simulink library "tcc"  (Simulink 8.1)
settings: Solver=ode1  StartTime=0.0  StopTime=Inf  FixedStep=0.001  RelTol=1e-3
PostLoadFcn:
  | , if any(exist('dsrtsu_mdlpostloadfcn', 'file') == [2, 3, 6]), try dsrtsu_mdlpostloadfcn('Execute', bdroot); catch fprintf('Error in PostLoadFcn (dsrtsu_mdlpostloadfcn) for model "%s":\n %s\n', bdroot, lasterr); end, end,
undefined symbols (not defined in the file or in its folder): KIFO_TTCDefault_s
libraries: simulink x4, hcu_lib x4
settings Model: DSRTSU_INTERNAL_RTI_VER=450  DSRTSU_INTERNAL_RTI_TYPE=rti1401  RTICANMMDATA=struct('GeneralSetupData',struct('modelroot','D:\PROJECTS\HAITEC\TAIWAN_HAITEC_SVN\trunk\AdasDragon\software\sw_development\arch\app\ifo','generalsettings',struct('filesettings',struct('destfolder',struct('Name','RTICANMM_FILES','Check',1),'buildfolder',struct('Name','.','Check',1),'AbsDestfolder',struct('Name','D:\PROJECTS\HAITEC\TAIWAN_HAITEC_SVN\trunk\AdasDragon\software\sw_development\arch\app\ifo\RTICANMM_FILES'),'AbsBuildfolder',struct('Name','D:\PROJECTS\HAITEC\TAIWAN_HAITEC_SVN\trunk\AdasDragon\software\sw_development\arch\app\ifo'))),'options',struct('addpaths',1,'rmpaths',1,'addtrcexclusion',logical(1),'cannavigator',struct('checkmonitoring',0),'show_usrtrc',0,'use_usrtrc',0),'advanced',struct('options',[1 1 1 1 1 1 1 1 1 1 1 1 1 1 1 1 1 1 1 1 1 1 1 1 1 1 1 1 1 1 1 1 1 1 1 1 1 1 1 1 1 1 1 1 1 1 1 1 1 1 1 1 1 1 1 1 1 1 1 1 1 1 1 1 1 1 1 1 1 1 1 1 1 1 1 1 1 1 1 1 1 1 1 1 1 1 1 1 1 1 1 1 1 1 1 1 1 1 1 1]),'MPSetup',{{}},'modelname','tcc','block','tcc'))  DSRTSU_INTERNAL_RTIFPGA=40  Creator=tescamilla  LastModifiedBy=tescamilla

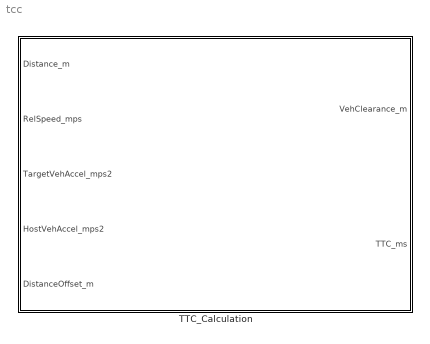
== system tcc ==
  TTC_Calculation : Subsystem

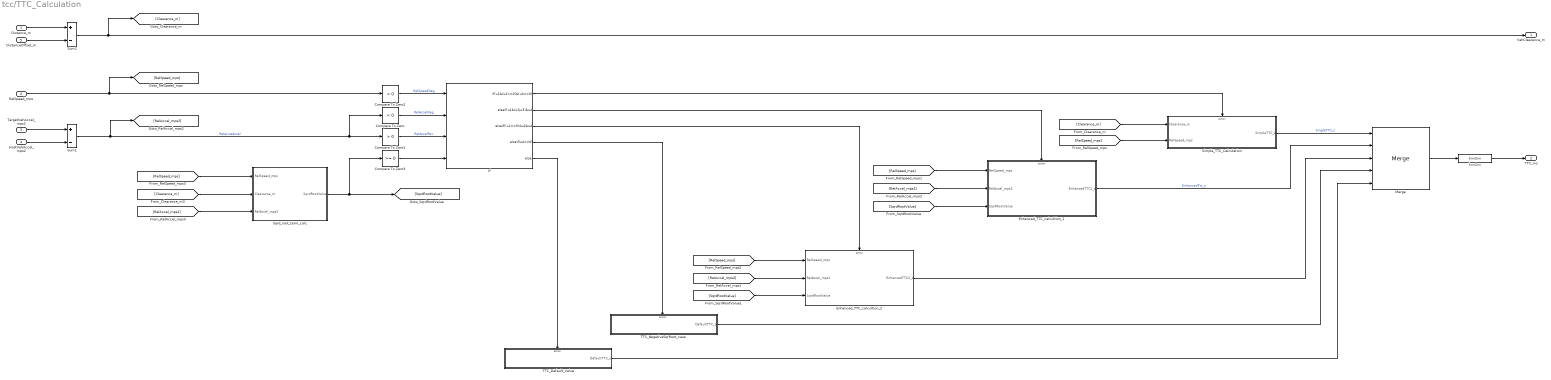
== system tcc/TTC_Calculation ==
  Distance_m : Inport
  RelSpeed_mps : Inport  Port=2
  TargetVehAccel_mps2 : Inport  Port=3
  HostVehAccel_mps2 : Inport  Port=4
  DistanceOffset_m : Inport  Port=5
  Compare To Zero : simulink/Logic and Bit Operations/Compare To Zero  relop=<  OutDataTypeStr=boolean
  Compare To Zero1 : simulink/Logic and Bit Operations/Compare To Zero  relop=>  OutDataTypeStr=boolean
  Compare To Zero2 : simulink/Logic and Bit Operations/Compare To Zero  relop=<  OutDataTypeStr=boolean
  Compare To Zero3 : simulink/Logic and Bit Operations/Compare To Zero  relop=>=  OutDataTypeStr=boolean
  Enhanced_TTC_calcultion_1 : Subsystem
  Enhanced_TTC_calcultion_2 : Subsystem
  If : If  NumInputs=4  IfExpression=u1&(u2==0)&(u3==0)  ElseIfExpressions=u1&(u2|u3)&u4,(u1==0)&u2&u4,u4==0
  Merge : Merge  Inputs=5  InitialOutput=KIFO_TTCDefault_s
  Simple_TTC_Calculation : Subsystem
  Sqrd_root_term_calc : Subsystem
  Sum1 : Sum  Inputs=+-
  Sum2 : Sum  Inputs=+-
  TTC_Default_Value : Subsystem
  TTC_NegativeSqrRoot_case : Subsystem
  kxx2xx : hcu_lib/kxx2xx
  VehClearance_m : Outport
  TTC_ms : Outport  Port=2
  wires:
  TargetVehAccel_mps2/1 -> Sum1/1
  HostVehAccel_mps2/1 -> Sum1/2
  Sum1/1 -> [RelAccel_mps2], Compare To Zero/1, Compare To Zero1/1  "RelativeAccel"
  RelSpeed_mps/1 -> [RelSpeed_mps], Compare To Zero2/1
  Compare To Zero2/1 -> If/1  "RelSpeedNeg"
  Compare To Zero/1 -> If/2  "RelAccelNeg"
  Compare To Zero1/1 -> If/3  "RelAccelPos"
  Distance_m/1 -> Sum2/1
  DistanceOffset_m/1 -> Sum2/2
  Sum2/1 -> [Clearance_m], VehClearance_m/1
  If/1 -> Simple_TTC_Calculation/Action
  If/2 -> Enhanced_TTC_calcultion_1/Action
  [Clearance_m] -> Simple_TTC_Calculation/1(Clearance_m)
  [RelSpeed_mps] -> Simple_TTC_Calculation/2(RelSpeed_mps)
  [RelSpeed_mps] -> Enhanced_TTC_calcultion_1/1(RelSpeed_mps)
  [RelAccel_mps2] -> Enhanced_TTC_calcultion_1/2(RelAccel_mps2)
  If/3 -> Enhanced_TTC_calcultion_2/Action
  [RelAccel_mps2] -> Enhanced_TTC_calcultion_2/2(RelAccel_mps2)
  [RelSpeed_mps] -> Enhanced_TTC_calcultion_2/1(RelSpeed_mps)
  If/5 -> TTC_Default_Value/Action
  Simple_TTC_Calculation/1(SimpleTTC_s) -> Merge/1  "SingleTTC_s"
  Enhanced_TTC_calcultion_1/1(EnhancedTTC1_s) -> Merge/2  "EnhancedTtc_s"
  Enhanced_TTC_calcultion_2/1(EnhancedTTC2_s) -> Merge/3
  TTC_Default_Value/1(DefaultTTC_s) -> Merge/5
  Merge/1 -> kxx2xx/1
  Compare To Zero3/1 -> If/4
  If/4 -> TTC_NegativeSqrRoot_case/Action
  TTC_NegativeSqrRoot_case/1(DefaultTTC_s) -> Merge/4
  [SqrdRootValue] -> Enhanced_TTC_calcultion_1/3(SqrdRootValue)
  [SqrdRootValue] -> Enhanced_TTC_calcultion_2/3(SqrdRootValue)
  Sqrd_root_term_calc/1(SqrdRootValue) -> Compare To Zero3/1, [SqrdRootValue]
  [RelSpeed_mps] -> Sqrd_root_term_calc/1(RelSpeed_mps)
  [Clearance_m] -> Sqrd_root_term_calc/2(Clearance_m)
  [RelAccel_mps2] -> Sqrd_root_term_calc/3(RelAccel_mps2)
  kxx2xx/1 -> TTC_ms/1

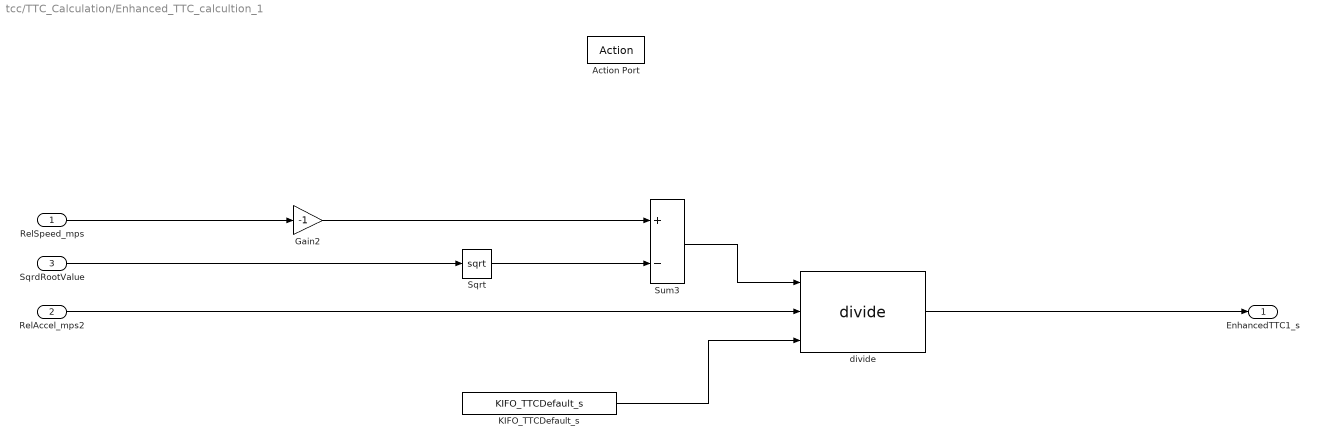
== system tcc/TTC_Calculation/Enhanced_TTC_calcultion_1 ==
  RelSpeed_mps : Inport
  RelAccel_mps2 : Inport  Port=2
  SqrdRootValue : Inport  Port=3
  Action Port : ActionPort  ActionType=elseif
  Gain2 : Gain  Gain=-1
  KIFO_TTCDefault_s : Constant  Value=KIFO_TTCDefault_s
  Sqrt : Sqrt  SaturateOnIntegerOverflow=on
  Sum3 : Sum  Inputs=+-
  divide : hcu_lib/divide
  EnhancedTTC1_s : Outport
  wires:
  divide/1 -> EnhancedTTC1_s/1
  KIFO_TTCDefault_s/1 -> divide/3
  Sum3/1 -> divide/1
  Sqrt/1 -> Sum3/2
  Gain2/1 -> Sum3/1
  SqrdRootValue/1 -> Sqrt/1
  RelSpeed_mps/1 -> Gain2/1
  RelAccel_mps2/1 -> divide/2

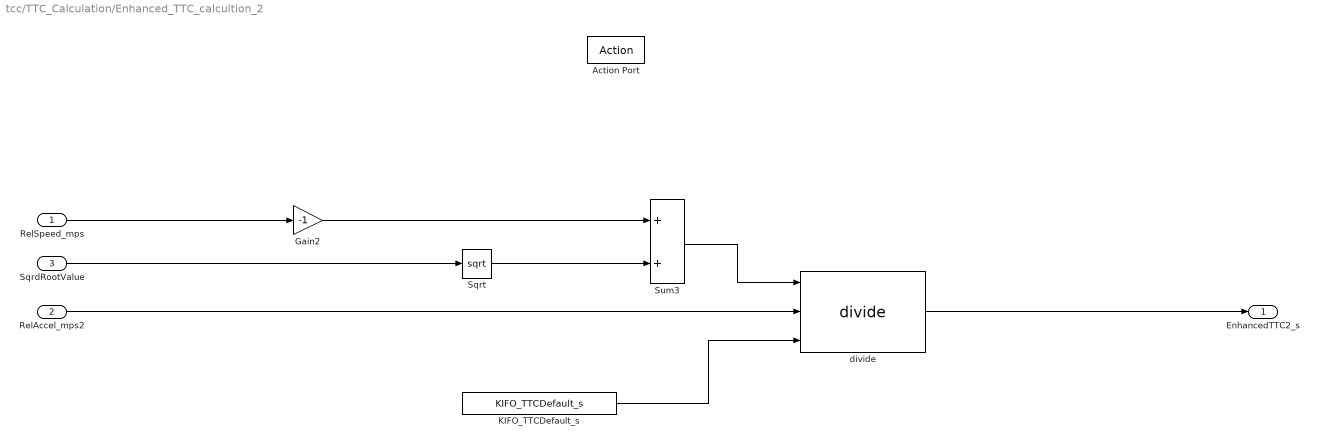
== system tcc/TTC_Calculation/Enhanced_TTC_calcultion_2 ==
  RelSpeed_mps : Inport
  RelAccel_mps2 : Inport  Port=2
  SqrdRootValue : Inport  Port=3
  Action Port : ActionPort  ActionType=elseif
  Gain2 : Gain  Gain=-1
  KIFO_TTCDefault_s : Constant  Value=KIFO_TTCDefault_s
  Sqrt : Sqrt  SaturateOnIntegerOverflow=on
  Sum3 : Sum
  divide : hcu_lib/divide
  EnhancedTTC2_s : Outport
  wires:
  RelAccel_mps2/1 -> divide/2
  RelSpeed_mps/1 -> Gain2/1
  SqrdRootValue/1 -> Sqrt/1
  Gain2/1 -> Sum3/1
  Sqrt/1 -> Sum3/2
  Sum3/1 -> divide/1
  KIFO_TTCDefault_s/1 -> divide/3
  divide/1 -> EnhancedTTC2_s/1

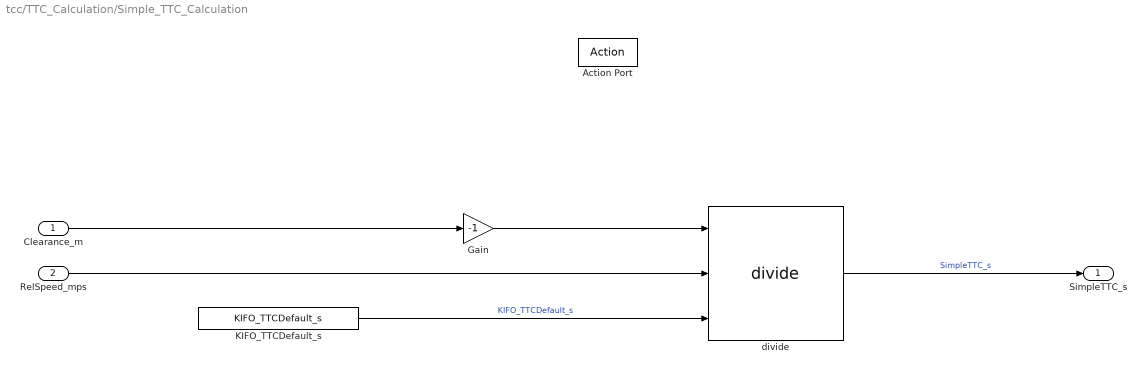
== system tcc/TTC_Calculation/Simple_TTC_Calculation ==
  Clearance_m : Inport
  RelSpeed_mps : Inport  Port=2
  Action Port : ActionPort  ActionType=then
  Gain : Gain  Gain=-1
  KIFO_TTCDefault_s : Constant  Value=KIFO_TTCDefault_s
  divide : hcu_lib/divide
  SimpleTTC_s : Outport
  wires:
  KIFO_TTCDefault_s/1 -> divide/3  "KIFO_TTCDefault_s"
  RelSpeed_mps/1 -> divide/2
  Clearance_m/1 -> Gain/1
  divide/1 -> SimpleTTC_s/1  "SimpleTTC_s"
  Gain/1 -> divide/1

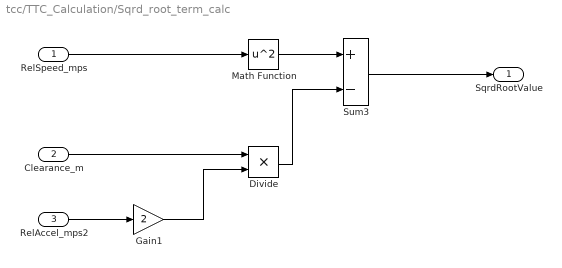
== system tcc/TTC_Calculation/Sqrd_root_term_calc ==
  RelSpeed_mps : Inport
  Clearance_m : Inport  Port=2
  RelAccel_mps2 : Inport  Port=3
  Divide : Product  Inputs=**
  Gain1 : Gain  Gain=2
  Math Function : Math  Operator=square  SaturateOnIntegerOverflow=on
  Sum3 : Sum  Inputs=+-
  SqrdRootValue : Outport
  wires:
  Sum3/1 -> SqrdRootValue/1
  Divide/1 -> Sum3/2
  RelSpeed_mps/1 -> Math Function/1
  Gain1/1 -> Divide/2
  RelAccel_mps2/1 -> Gain1/1
  Math Function/1 -> Sum3/1
  Clearance_m/1 -> Divide/1

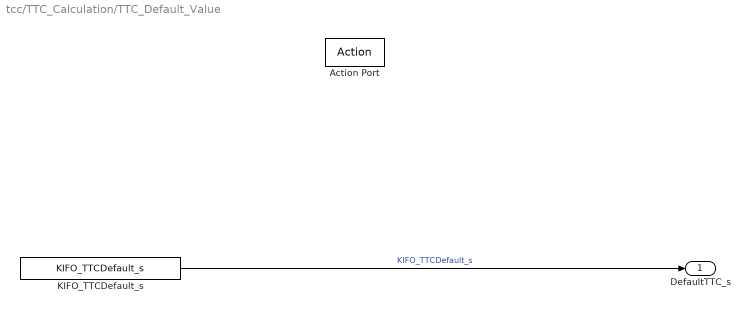
== system tcc/TTC_Calculation/TTC_Default_Value ==
  Action Port : ActionPort  ActionType=else
  KIFO_TTCDefault_s : Constant  Value=KIFO_TTCDefault_s
  DefaultTTC_s : Outport
  wires:
  KIFO_TTCDefault_s/1 -> DefaultTTC_s/1  "KIFO_TTCDefault_s"

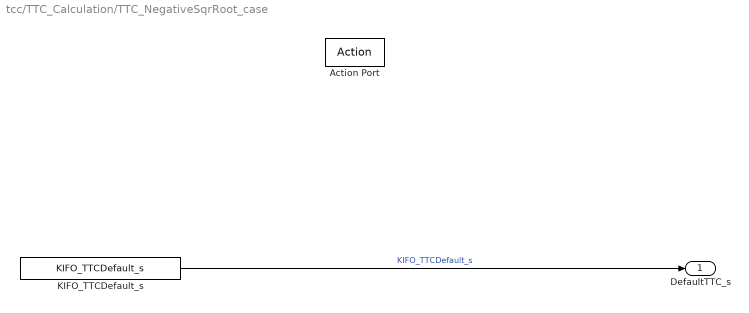
== system tcc/TTC_Calculation/TTC_NegativeSqrRoot_case ==
  Action Port : ActionPort  ActionType=elseif
  KIFO_TTCDefault_s : Constant  Value=KIFO_TTCDefault_s
  DefaultTTC_s : Outport
  wires:
  KIFO_TTCDefault_s/1 -> DefaultTTC_s/1  "KIFO_TTCDefault_s"
